simulink model "chap05"  (R2021a)
settings: Solver=FixedStepDiscrete  StartTime=0.0  StopTime=inf  FixedStep=0.001  RelTol=1e-3
undefined symbols (not defined in the file): DiscIntNeverNeededParam, Header, Pose, X, Y, Z
libraries: robotlib x31
(part 8 of 9)

== system chap05/Subsystem16/Subsystem2/Subsystem9/Subsystem ==
  switch : Inport
  zt3 : Inport  Port=2
  Constant4 : Constant  Value=0
  Discrete-Time Integrator : DiscreteIntegrator  SampleTime=-1  UpperSaturationLimit=100  LowerSaturationLimit=-100  ICPrevOutput=DiscIntNeverNeededParam  ICPrevScaledInput=DiscIntNeverNeededParam
  Logical Operator : Logic  AllPortsSameDT=off  OutDataTypeStr=boolean
  MATLAB Function : MATLAB Function  TreatAsAtomicUnit=on
  Relational Operator : RelationalOperator  Operator===  OutDataTypeStr=boolean  RndMeth=Simplest
  Saturation1 : Saturate  UpperLimit=0.25  LowerLimit=-0.25
  Sign : Signum
  Sign1 : Signum
  Subsystem : Subsystem
      settings: PortSchema="{\"entries\":[{\"content\":{\"sides\":[{\"content\":{\"connectorIds\":[\"In1\"]},\"type\":\"ConnectorPlacement.EquallySpacedRectSide\",\"uuid\":\"50b1559e-7173-4ba8-93e6-314f6d9df527\"},{\"content\":{\"connectorIds\":[\"Out1\"],\"side\":\"RIGHT\"},\"type\":\"ConnectorPlacement.EquallySpacedRectSide\",\"uuid\":\"be527bac-0bcc-4faf-a185-0382edae0189\"},{\"content\":{\"connectorIds\":[\"In2\"],\"side\":\"TOP\"},\"type\":\"ConnectorPlacement.EquallySpacedRectSide\",\"uuid\":\"4c8ef68d-7cf5-4d15-9758-89dbc1169805\"}]},\"type\":\"ConnectorPlacement.EquallySpacedConnector\",\"uuid\":\"3c2ee67b-c3c9-431a-8107-6d5cd22b236e\"}],\"packageUris\":[\"http://schema.mathworks.com/mf0/Connector/R2020b\"],\"version\":\"1.0\"}"
  Switch : Switch  Criteria=u2 > Threshold
  Out1 : Outport
  wires:
  zt3/1 -> Subsystem/1(zt3)
  switch/1 -> Subsystem/2(switch)
  Switch/1 -> Discrete-Time Integrator/1
  Logical Operator/1 -> Switch/2
  Sign/1 -> Relational Operator/2
  Discrete-Time Integrator/1 -> Saturation1/1, Sign/1, MATLAB Function/1(u1)
  Saturation1/1 -> MATLAB Function/2(u2), Out1/1
  Subsystem/1(Out1) -> Switch/3, Sign1/1
  Sign1/1 -> Relational Operator/1
  Constant4/1 -> Switch/1
  Relational Operator/1 -> Logical Operator/2
  MATLAB Function/1(y) -> Logical Operator/1

== system chap05/Subsystem16/Subsystem3/Subsystem11/Subsystem ==
  switch : Inport
  zt3 : Inport  Port=2
  Constant4 : Constant  Value=0
  Discrete-Time Integrator : DiscreteIntegrator  SampleTime=-1  UpperSaturationLimit=100  LowerSaturationLimit=-100  ICPrevOutput=DiscIntNeverNeededParam  ICPrevScaledInput=DiscIntNeverNeededParam
  Logical Operator : Logic  AllPortsSameDT=off  OutDataTypeStr=boolean
  MATLAB Function : MATLAB Function  TreatAsAtomicUnit=on
  Relational Operator : RelationalOperator  Operator===  OutDataTypeStr=boolean  RndMeth=Simplest
  Saturation1 : Saturate  UpperLimit=0.25  LowerLimit=-0.25
  Sign : Signum
  Sign1 : Signum
  Subsystem : Subsystem
      settings: PortSchema="{\"entries\":[{\"content\":{\"sides\":[{\"content\":{\"connectorIds\":[\"In1\"]},\"type\":\"ConnectorPlacement.EquallySpacedRectSide\",\"uuid\":\"50b1559e-7173-4ba8-93e6-314f6d9df527\"},{\"content\":{\"connectorIds\":[\"Out1\"],\"side\":\"RIGHT\"},\"type\":\"ConnectorPlacement.EquallySpacedRectSide\",\"uuid\":\"be527bac-0bcc-4faf-a185-0382edae0189\"},{\"content\":{\"connectorIds\":[\"In2\"],\"side\":\"TOP\"},\"type\":\"ConnectorPlacement.EquallySpacedRectSide\",\"uuid\":\"4c8ef68d-7cf5-4d15-9758-89dbc1169805\"}]},\"type\":\"ConnectorPlacement.EquallySpacedConnector\",\"uuid\":\"3c2ee67b-c3c9-431a-8107-6d5cd22b236e\"}],\"packageUris\":[\"http://schema.mathworks.com/mf0/Connector/R2020b\"],\"version\":\"1.0\"}"
  Switch : Switch  Criteria=u2 > Threshold
  Out1 : Outport
  wires:
  MATLAB Function/1(y) -> Logical Operator/1
  Relational Operator/1 -> Logical Operator/2
  Constant4/1 -> Switch/1
  Sign1/1 -> Relational Operator/1
  Subsystem/1(Out1) -> Sign1/1, Switch/3
  Saturation1/1 -> Out1/1, MATLAB Function/2(u2)
  Discrete-Time Integrator/1 -> Saturation1/1, MATLAB Function/1(u1), Sign/1
  Sign/1 -> Relational Operator/2
  Logical Operator/1 -> Switch/2
  Switch/1 -> Discrete-Time Integrator/1
  zt3/1 -> Subsystem/1(zt3)
  switch/1 -> Subsystem/2(switch)

== system chap05/Subsystem16/Subsystem3/Subsystem3/Subsystem ==
  e1 : Inport
  k3 : Inport  Port=2
  k4 : Inport  Port=3
  Add : Sum
  Constant3 : Constant  Value=-1
  Constant4 : Constant  Value=-1
  Discrete-Time Integrator1 : DiscreteIntegrator  SampleTime=-1  ICPrevOutput=DiscIntNeverNeededParam  ICPrevScaledInput=DiscIntNeverNeededParam
  Divide : Product  Inputs=*/
  MATLAB Function : MATLAB Function  TreatAsAtomicUnit=on
  Product3 : Product  Inputs=3
  Product5 : Product  Inputs=3
  z2 : Outport
  wires:
  Constant4/1 -> Product5/1
  Product5/1 -> Add/2
  Discrete-Time Integrator1/1 -> z2/1
  k3/1 -> Product3/3
  k4/1 -> Product5/3
  Divide/1 -> Add/1
  Add/1 -> Discrete-Time Integrator1/1
  Constant3/1 -> Product3/1
  e1/1 -> Product5/2, MATLAB Function/1(u), Product3/2
  MATLAB Function/1(y) -> Divide/2
  Product3/1 -> Divide/1

== system chap05/Subsystem16/Subsystem3/Subsystem3/Subsystem1 ==
  e1 : Inport
  k1 : Inport  Port=2
  Constant : Constant  Value=-1
  Divide : Product  Inputs=*/
  MATLAB Function : MATLAB Function  TreatAsAtomicUnit=on
  Product : Product  Inputs=3
  Out1 : Outport
  wires:
  e1/1 -> Product/2, MATLAB Function/1(u)
  Divide/1 -> Out1/1
  Constant/1 -> Product/1
  k1/1 -> Product/3
  MATLAB Function/1(y) -> Divide/2
  Product/1 -> Divide/1

== system chap05/Subsystem16/Subsystem3/Subsystem3/Subsystem2 ==
  e1 : Inport
  switch : Inport  Port=2
  Constant1 : Constant  Value=0.1
  MATLAB Function : MATLAB Function  TreatAsAtomicUnit=on
  Product{,1..3,6} (5 alike) : Product
  Sqrt : Sqrt  SaturateOnIntegerOverflow=on
  Square : Math  Operator=square  SaturateOnIntegerOverflow=on
  Subsystem : Subsystem
      settings: PortSchema="{\"entries\":[{\"content\":{\"sides\":[{\"content\":{\"connectorIds\":[\"In1\"]},\"type\":\"ConnectorPlacement.EquallySpacedRectSide\",\"uuid\":\"12a3f2f0-a297-420d-b26a-5f62088d5514\"},{\"content\":{\"connectorIds\":[\"Out1\"],\"side\":\"RIGHT\"},\"type\":\"ConnectorPlacement.EquallySpacedRectSide\",\"uuid\":\"62e35448-e0a3-4495-a6db-77deef7aa7b4\"},{\"content\":{\"connectorIds\":[\"In2\"],\"side\":\"TOP\"},\"type\":\"ConnectorPlacement.EquallySpacedRectSide\",\"uuid\":\"3e6c604a-b26b-4ac2-9bdc-2cdec7247e53\"}]},\"type\":\"ConnectorPlacement.EquallySpacedConnector\",\"uuid\":\"6331fe4a-63c7-4003-9b0d-be968a8635fa\"}],\"packageUris\":[\"http://schema.mathworks.com/mf0/Connector/R2020b\"],\"version\":\"1.0\"}"
  Subtract2 : Sum  Inputs=+-
  c1 : Constant  Value=0.1
  c2 : Constant  Value=0.1
  c3 : Constant  Value=0.3
  c4 : Constant  Value=0.3
  k1 : Outport
  k2 : Outport  Port=2
  k3 : Outport  Port=3
  k4 : Outport  Port=4
  wires:
  c2/1 -> Product/2
  Product/1 -> k2/1
  c3/1 -> Product1/1
  Product1/1 -> k3/1
  c4/1 -> Product2/1
  Product2/1 -> k4/1
  c1/1 -> Product3/2
  Product3/1 -> k1/1
  Sqrt/1 -> Product3/1
  Square/1 -> Product2/2
  e1/1 -> MATLAB Function/1(u)
  Product6/1 -> Subtract2/2
  MATLAB Function/1(y) -> Subtract2/1
  Subtract2/1 -> Subsystem/1(In1)
  Constant1/1 -> Product6/1
  switch/1 -> Subsystem/2(switch)
  Subsystem/1(Out1) -> Product6/2, Sqrt/1, Product1/2, Square/1, Product/1

== system chap05/Subsystem16/Subsystem3/Subsystem3/Subsystem3 ==
  e1 : Inport
  k2 : Inport  Port=2
  Constant2 : Constant  Value=-1
  Product2 : Product  Inputs=3
  Out1 : Outport
  wires:
  Product2/1 -> Out1/1
  e1/1 -> Product2/2
  k2/1 -> Product2/3
  Constant2/1 -> Product2/1

== system chap05/Subsystem16/Subsystem3/Subsystem4/Subsystem ==
  switch : Inport
  zt3 : Inport  Port=2
  Constant4 : Constant  Value=0
  Discrete-Time Integrator : DiscreteIntegrator  SampleTime=-1  UpperSaturationLimit=100  LowerSaturationLimit=-100  ICPrevOutput=DiscIntNeverNeededParam  ICPrevScaledInput=DiscIntNeverNeededParam
  Logical Operator : Logic  AllPortsSameDT=off  OutDataTypeStr=boolean
  MATLAB Function : MATLAB Function  TreatAsAtomicUnit=on
  Relational Operator : RelationalOperator  Operator===  OutDataTypeStr=boolean  RndMeth=Simplest
  Saturation1 : Saturate  UpperLimit=0.25  LowerLimit=-0.25
  Sign : Signum
  Sign1 : Signum
  Subsystem : Subsystem
      settings: PortSchema="{\"entries\":[{\"content\":{\"sides\":[{\"content\":{\"connectorIds\":[\"In1\"]},\"type\":\"ConnectorPlacement.EquallySpacedRectSide\",\"uuid\":\"50b1559e-7173-4ba8-93e6-314f6d9df527\"},{\"content\":{\"connectorIds\":[\"Out1\"],\"side\":\"RIGHT\"},\"type\":\"ConnectorPlacement.EquallySpacedRectSide\",\"uuid\":\"be527bac-0bcc-4faf-a185-0382edae0189\"},{\"content\":{\"connectorIds\":[\"In2\"],\"side\":\"TOP\"},\"type\":\"ConnectorPlacement.EquallySpacedRectSide\",\"uuid\":\"4c8ef68d-7cf5-4d15-9758-89dbc1169805\"}]},\"type\":\"ConnectorPlacement.EquallySpacedConnector\",\"uuid\":\"3c2ee67b-c3c9-431a-8107-6d5cd22b236e\"}],\"packageUris\":[\"http://schema.mathworks.com/mf0/Connector/R2020b\"],\"version\":\"1.0\"}"
  Switch : Switch  Criteria=u2 > Threshold
  Out1 : Outport
  wires:
  MATLAB Function/1(y) -> Logical Operator/1
  Relational Operator/1 -> Logical Operator/2
  Constant4/1 -> Switch/1
  Sign1/1 -> Relational Operator/1
  Subsystem/1(Out1) -> Sign1/1, Switch/3
  Saturation1/1 -> Out1/1, MATLAB Function/2(u2)
  Discrete-Time Integrator/1 -> Saturation1/1, MATLAB Function/1(u1), Sign/1
  Sign/1 -> Relational Operator/2
  Logical Operator/1 -> Switch/2
  Switch/1 -> Discrete-Time Integrator/1
  zt3/1 -> Subsystem/1(zt3)
  switch/1 -> Subsystem/2(switch)

== system chap05/Subsystem16/Subsystem3/Subsystem8/Subsystem ==
  In1 : Inport
  switch : Inport  Port=2
  Constant4 : Constant  Value=0
  Switch1 : Switch  Criteria=u2 > Threshold
  Out1 : Outport
  wires:
  In1/1 -> Switch1/1
  Switch1/1 -> Out1/1
  switch/1 -> Switch1/2
  Constant4/1 -> Switch1/3

== system chap05/Subsystem16/Subsystem3/Subsystem8/Subsystem1 ==
  In1 : Inport
  switch : Inport  Port=2
  Constant4 : Constant  Value=0
  Switch1 : Switch  Criteria=u2 > Threshold
  Out1 : Outport
  wires:
  Constant4/1 -> Switch1/3
  switch/1 -> Switch1/2
  Switch1/1 -> Out1/1
  In1/1 -> Switch1/1

== system chap05/Subsystem16/Subsystem3/Subsystem8/Subsystem2 ==
  In1 : Inport
  switch : Inport  Port=2
  Constant4 : Constant  Value=0
  Switch1 : Switch  Criteria=u2 > Threshold
  Out1 : Outport
  wires:
  In1/1 -> Switch1/1
  Switch1/1 -> Out1/1
  switch/1 -> Switch1/2
  Constant4/1 -> Switch1/3

== system chap05/Subsystem16/Subsystem3/Subsystem9/Subsystem ==
  switch : Inport
  zt3 : Inport  Port=2
  Constant4 : Constant  Value=0
  Discrete-Time Integrator : DiscreteIntegrator  SampleTime=-1  UpperSaturationLimit=100  LowerSaturationLimit=-100  ICPrevOutput=DiscIntNeverNeededParam  ICPrevScaledInput=DiscIntNeverNeededParam
  Logical Operator : Logic  AllPortsSameDT=off  OutDataTypeStr=boolean
  MATLAB Function : MATLAB Function  TreatAsAtomicUnit=on
  Relational Operator : RelationalOperator  Operator===  OutDataTypeStr=boolean  RndMeth=Simplest
  Saturation1 : Saturate  UpperLimit=0.25  LowerLimit=-0.25
  Sign : Signum
  Sign1 : Signum
  Subsystem : Subsystem
      settings: PortSchema="{\"entries\":[{\"content\":{\"sides\":[{\"content\":{\"connectorIds\":[\"In1\"]},\"type\":\"ConnectorPlacement.EquallySpacedRectSide\",\"uuid\":\"50b1559e-7173-4ba8-93e6-314f6d9df527\"},{\"content\":{\"connectorIds\":[\"Out1\"],\"side\":\"RIGHT\"},\"type\":\"ConnectorPlacement.EquallySpacedRectSide\",\"uuid\":\"be527bac-0bcc-4faf-a185-0382edae0189\"},{\"content\":{\"connectorIds\":[\"In2\"],\"side\":\"TOP\"},\"type\":\"ConnectorPlacement.EquallySpacedRectSide\",\"uuid\":\"4c8ef68d-7cf5-4d15-9758-89dbc1169805\"}]},\"type\":\"ConnectorPlacement.EquallySpacedConnector\",\"uuid\":\"3c2ee67b-c3c9-431a-8107-6d5cd22b236e\"}],\"packageUris\":[\"http://schema.mathworks.com/mf0/Connector/R2020b\"],\"version\":\"1.0\"}"
  Switch : Switch  Criteria=u2 > Threshold
  Out1 : Outport
  wires:
  zt3/1 -> Subsystem/1(zt3)
  switch/1 -> Subsystem/2(switch)
  Switch/1 -> Discrete-Time Integrator/1
  Logical Operator/1 -> Switch/2
  Sign/1 -> Relational Operator/2
  Discrete-Time Integrator/1 -> Saturation1/1, Sign/1, MATLAB Function/1(u1)
  Saturation1/1 -> MATLAB Function/2(u2), Out1/1
  Subsystem/1(Out1) -> Switch/3, Sign1/1
  Sign1/1 -> Relational Operator/1
  Constant4/1 -> Switch/1
  Relational Operator/1 -> Logical Operator/2
  MATLAB Function/1(y) -> Logical Operator/1

== system chap05/Subsystem16/Subsystem5/Subsystem11/Subsystem ==
  switch : Inport
  zt3 : Inport  Port=2
  Constant4 : Constant  Value=0
  Discrete-Time Integrator : DiscreteIntegrator  SampleTime=-1  UpperSaturationLimit=100  LowerSaturationLimit=-100  ICPrevOutput=DiscIntNeverNeededParam  ICPrevScaledInput=DiscIntNeverNeededParam
  Logical Operator : Logic  AllPortsSameDT=off  OutDataTypeStr=boolean
  MATLAB Function : MATLAB Function  TreatAsAtomicUnit=on
  Relational Operator : RelationalOperator  Operator===  OutDataTypeStr=boolean  RndMeth=Simplest
  Saturation1 : Saturate  UpperLimit=0.25  LowerLimit=-0.25
  Sign : Signum
  Sign1 : Signum
  Subsystem : Subsystem
      settings: PortSchema="{\"entries\":[{\"content\":{\"sides\":[{\"content\":{\"connectorIds\":[\"In1\"]},\"type\":\"ConnectorPlacement.EquallySpacedRectSide\",\"uuid\":\"50b1559e-7173-4ba8-93e6-314f6d9df527\"},{\"content\":{\"connectorIds\":[\"Out1\"],\"side\":\"RIGHT\"},\"type\":\"ConnectorPlacement.EquallySpacedRectSide\",\"uuid\":\"be527bac-0bcc-4faf-a185-0382edae0189\"},{\"content\":{\"connectorIds\":[\"In2\"],\"side\":\"TOP\"},\"type\":\"ConnectorPlacement.EquallySpacedRectSide\",\"uuid\":\"4c8ef68d-7cf5-4d15-9758-89dbc1169805\"}]},\"type\":\"ConnectorPlacement.EquallySpacedConnector\",\"uuid\":\"3c2ee67b-c3c9-431a-8107-6d5cd22b236e\"}],\"packageUris\":[\"http://schema.mathworks.com/mf0/Connector/R2020b\"],\"version\":\"1.0\"}"
  Switch : Switch  Criteria=u2 > Threshold
  Out1 : Outport
  wires:
  MATLAB Function/1(y) -> Logical Operator/1
  Relational Operator/1 -> Logical Operator/2
  Constant4/1 -> Switch/1
  Sign1/1 -> Relational Operator/1
  Subsystem/1(Out1) -> Sign1/1, Switch/3
  Saturation1/1 -> Out1/1, MATLAB Function/2(u2)
  Discrete-Time Integrator/1 -> Saturation1/1, MATLAB Function/1(u1), Sign/1
  Sign/1 -> Relational Operator/2
  Logical Operator/1 -> Switch/2
  Switch/1 -> Discrete-Time Integrator/1
  zt3/1 -> Subsystem/1(zt3)
  switch/1 -> Subsystem/2(switch)

== system chap05/Subsystem16/Subsystem5/Subsystem3/Subsystem ==
  e1 : Inport
  k3 : Inport  Port=2
  k4 : Inport  Port=3
  Add : Sum
  Constant3 : Constant  Value=-1
  Constant4 : Constant  Value=-1
  Discrete-Time Integrator1 : DiscreteIntegrator  SampleTime=-1  ICPrevOutput=DiscIntNeverNeededParam  ICPrevScaledInput=DiscIntNeverNeededParam
  Divide : Product  Inputs=*/
  MATLAB Function : MATLAB Function  TreatAsAtomicUnit=on
  Product3 : Product  Inputs=3
  Product5 : Product  Inputs=3
  z2 : Outport
  wires:
  Constant4/1 -> Product5/1
  Product5/1 -> Add/2
  Discrete-Time Integrator1/1 -> z2/1
  k3/1 -> Product3/3
  k4/1 -> Product5/3
  Divide/1 -> Add/1
  Add/1 -> Discrete-Time Integrator1/1
  Constant3/1 -> Product3/1
  e1/1 -> Product5/2, MATLAB Function/1(u), Product3/2
  MATLAB Function/1(y) -> Divide/2
  Product3/1 -> Divide/1

== system chap05/Subsystem16/Subsystem5/Subsystem3/Subsystem1 ==
  e1 : Inport
  k1 : Inport  Port=2
  Constant : Constant  Value=-1
  Divide : Product  Inputs=*/
  MATLAB Function : MATLAB Function  TreatAsAtomicUnit=on
  Product : Product  Inputs=3
  Out1 : Outport
  wires:
  e1/1 -> Product/2, MATLAB Function/1(u)
  Divide/1 -> Out1/1
  Constant/1 -> Product/1
  k1/1 -> Product/3
  MATLAB Function/1(y) -> Divide/2
  Product/1 -> Divide/1

== system chap05/Subsystem16/Subsystem5/Subsystem3/Subsystem2 ==
  e1 : Inport
  switch : Inport  Port=2
  Constant1 : Constant  Value=0.1
  MATLAB Function : MATLAB Function  TreatAsAtomicUnit=on
  Product{,1..3,6} (5 alike) : Product
  Sqrt : Sqrt  SaturateOnIntegerOverflow=on
  Square : Math  Operator=square  SaturateOnIntegerOverflow=on
  Subsystem : Subsystem
      settings: PortSchema="{\"entries\":[{\"content\":{\"sides\":[{\"content\":{\"connectorIds\":[\"In1\"]},\"type\":\"ConnectorPlacement.EquallySpacedRectSide\",\"uuid\":\"12a3f2f0-a297-420d-b26a-5f62088d5514\"},{\"content\":{\"connectorIds\":[\"Out1\"],\"side\":\"RIGHT\"},\"type\":\"ConnectorPlacement.EquallySpacedRectSide\",\"uuid\":\"62e35448-e0a3-4495-a6db-77deef7aa7b4\"},{\"content\":{\"connectorIds\":[\"In2\"],\"side\":\"TOP\"},\"type\":\"ConnectorPlacement.EquallySpacedRectSide\",\"uuid\":\"3e6c604a-b26b-4ac2-9bdc-2cdec7247e53\"}]},\"type\":\"ConnectorPlacement.EquallySpacedConnector\",\"uuid\":\"6331fe4a-63c7-4003-9b0d-be968a8635fa\"}],\"packageUris\":[\"http://schema.mathworks.com/mf0/Connector/R2020b\"],\"version\":\"1.0\"}"
  Subtract2 : Sum  Inputs=+-
  c1 : Constant  Value=0.1
  c2 : Constant  Value=0.1
  c3 : Constant  Value=0.3
  c4 : Constant  Value=0.3
  k1 : Outport
  k2 : Outport  Port=2
  k3 : Outport  Port=3
  k4 : Outport  Port=4
  wires:
  c2/1 -> Product/2
  Product/1 -> k2/1
  c3/1 -> Product1/1
  Product1/1 -> k3/1
  c4/1 -> Product2/1
  Product2/1 -> k4/1
  c1/1 -> Product3/2
  Product3/1 -> k1/1
  Sqrt/1 -> Product3/1
  Square/1 -> Product2/2
  e1/1 -> MATLAB Function/1(u)
  Product6/1 -> Subtract2/2
  MATLAB Function/1(y) -> Subtract2/1
  Subtract2/1 -> Subsystem/1(In1)
  Constant1/1 -> Product6/1
  switch/1 -> Subsystem/2(switch)
  Subsystem/1(Out1) -> Product6/2, Sqrt/1, Product1/2, Square/1, Product/1

== system chap05/Subsystem16/Subsystem5/Subsystem3/Subsystem3 ==
  e1 : Inport
  k2 : Inport  Port=2
  Constant2 : Constant  Value=-1
  Product2 : Product  Inputs=3
  Out1 : Outport
  wires:
  Product2/1 -> Out1/1
  e1/1 -> Product2/2
  k2/1 -> Product2/3
  Constant2/1 -> Product2/1

== system chap05/Subsystem16/Subsystem5/Subsystem4/Subsystem ==
  switch : Inport
  zt3 : Inport  Port=2
  Constant4 : Constant  Value=0
  Discrete-Time Integrator : DiscreteIntegrator  SampleTime=-1  UpperSaturationLimit=100  LowerSaturationLimit=-100  ICPrevOutput=DiscIntNeverNeededParam  ICPrevScaledInput=DiscIntNeverNeededParam
  Logical Operator : Logic  AllPortsSameDT=off  OutDataTypeStr=boolean
  MATLAB Function : MATLAB Function  TreatAsAtomicUnit=on
  Relational Operator : RelationalOperator  Operator===  OutDataTypeStr=boolean  RndMeth=Simplest
  Saturation1 : Saturate  UpperLimit=0.25  LowerLimit=-0.25
  Sign : Signum
  Sign1 : Signum
  Subsystem : Subsystem
      settings: PortSchema="{\"entries\":[{\"content\":{\"sides\":[{\"content\":{\"connectorIds\":[\"In1\"]},\"type\":\"ConnectorPlacement.EquallySpacedRectSide\",\"uuid\":\"50b1559e-7173-4ba8-93e6-314f6d9df527\"},{\"content\":{\"connectorIds\":[\"Out1\"],\"side\":\"RIGHT\"},\"type\":\"ConnectorPlacement.EquallySpacedRectSide\",\"uuid\":\"be527bac-0bcc-4faf-a185-0382edae0189\"},{\"content\":{\"connectorIds\":[\"In2\"],\"side\":\"TOP\"},\"type\":\"ConnectorPlacement.EquallySpacedRectSide\",\"uuid\":\"4c8ef68d-7cf5-4d15-9758-89dbc1169805\"}]},\"type\":\"ConnectorPlacement.EquallySpacedConnector\",\"uuid\":\"3c2ee67b-c3c9-431a-8107-6d5cd22b236e\"}],\"packageUris\":[\"http://schema.mathworks.com/mf0/Connector/R2020b\"],\"version\":\"1.0\"}"
  Switch : Switch  Criteria=u2 > Threshold
  Out1 : Outport
  wires:
  MATLAB Function/1(y) -> Logical Operator/1
  Relational Operator/1 -> Logical Operator/2
  Constant4/1 -> Switch/1
  Sign1/1 -> Relational Operator/1
  Subsystem/1(Out1) -> Sign1/1, Switch/3
  Saturation1/1 -> Out1/1, MATLAB Function/2(u2)
  Discrete-Time Integrator/1 -> Saturation1/1, MATLAB Function/1(u1), Sign/1
  Sign/1 -> Relational Operator/2
  Logical Operator/1 -> Switch/2
  Switch/1 -> Discrete-Time Integrator/1
  zt3/1 -> Subsystem/1(zt3)
  switch/1 -> Subsystem/2(switch)

== system chap05/Subsystem16/Subsystem5/Subsystem7/Subsystem ==
  In1 : Inport
  switch : Inport  Port=2
  Constant4 : Constant  Value=0
  Switch1 : Switch  Criteria=u2 > Threshold
  Out1 : Outport
  wires:
  In1/1 -> Switch1/1
  Switch1/1 -> Out1/1
  switch/1 -> Switch1/2
  Constant4/1 -> Switch1/3

== system chap05/Subsystem16/Subsystem5/Subsystem7/Subsystem1 ==
  In1 : Inport
  switch : Inport  Port=2
  Constant4 : Constant  Value=0
  Switch1 : Switch  Criteria=u2 > Threshold
  Out1 : Outport
  wires:
  Constant4/1 -> Switch1/3
  switch/1 -> Switch1/2
  Switch1/1 -> Out1/1
  In1/1 -> Switch1/1

== system chap05/Subsystem16/Subsystem5/Subsystem7/Subsystem2 ==
  In1 : Inport
  switch : Inport  Port=2
  Constant4 : Constant  Value=0
  Switch1 : Switch  Criteria=u2 > Threshold
  Out1 : Outport
  wires:
  In1/1 -> Switch1/1
  Switch1/1 -> Out1/1
  switch/1 -> Switch1/2
  Constant4/1 -> Switch1/3

== system chap05/Subsystem16/Subsystem5/Subsystem9/Subsystem ==
  switch : Inport
  zt3 : Inport  Port=2
  Constant4 : Constant  Value=0
  Discrete-Time Integrator : DiscreteIntegrator  SampleTime=-1  UpperSaturationLimit=100  LowerSaturationLimit=-100  ICPrevOutput=DiscIntNeverNeededParam  ICPrevScaledInput=DiscIntNeverNeededParam
  Logical Operator : Logic  AllPortsSameDT=off  OutDataTypeStr=boolean
  MATLAB Function : MATLAB Function  TreatAsAtomicUnit=on
  Relational Operator : RelationalOperator  Operator===  OutDataTypeStr=boolean  RndMeth=Simplest
  Saturation1 : Saturate  UpperLimit=0.25  LowerLimit=-0.25
  Sign : Signum
  Sign1 : Signum
  Subsystem : Subsystem
      settings: PortSchema="{\"entries\":[{\"content\":{\"sides\":[{\"content\":{\"connectorIds\":[\"In1\"]},\"type\":\"ConnectorPlacement.EquallySpacedRectSide\",\"uuid\":\"50b1559e-7173-4ba8-93e6-314f6d9df527\"},{\"content\":{\"connectorIds\":[\"Out1\"],\"side\":\"RIGHT\"},\"type\":\"ConnectorPlacement.EquallySpacedRectSide\",\"uuid\":\"be527bac-0bcc-4faf-a185-0382edae0189\"},{\"content\":{\"connectorIds\":[\"In2\"],\"side\":\"TOP\"},\"type\":\"ConnectorPlacement.EquallySpacedRectSide\",\"uuid\":\"4c8ef68d-7cf5-4d15-9758-89dbc1169805\"}]},\"type\":\"ConnectorPlacement.EquallySpacedConnector\",\"uuid\":\"3c2ee67b-c3c9-431a-8107-6d5cd22b236e\"}],\"packageUris\":[\"http://schema.mathworks.com/mf0/Connector/R2020b\"],\"version\":\"1.0\"}"
  Switch : Switch  Criteria=u2 > Threshold
  Out1 : Outport
  wires:
  zt3/1 -> Subsystem/1(zt3)
  switch/1 -> Subsystem/2(switch)
  Switch/1 -> Discrete-Time Integrator/1
  Logical Operator/1 -> Switch/2
  Sign/1 -> Relational Operator/2
  Discrete-Time Integrator/1 -> Saturation1/1, Sign/1, MATLAB Function/1(u1)
  Saturation1/1 -> MATLAB Function/2(u2), Out1/1
  Subsystem/1(Out1) -> Switch/3, Sign1/1
  Sign1/1 -> Relational Operator/1
  Constant4/1 -> Switch/1
  Relational Operator/1 -> Logical Operator/2
  MATLAB Function/1(y) -> Logical Operator/1

== system chap05/Subsystem16/Subsystem6/Subsystem3/Subsystem ==
  e1 : Inport
  k3 : Inport  Port=2
  k4 : Inport  Port=3
  Add : Sum
  Constant3 : Constant  Value=-1
  Constant4 : Constant  Value=-1
  Discrete-Time Integrator1 : DiscreteIntegrator  SampleTime=-1  ICPrevOutput=DiscIntNeverNeededParam  ICPrevScaledInput=DiscIntNeverNeededParam
  Divide : Product  Inputs=*/
  MATLAB Function : MATLAB Function  TreatAsAtomicUnit=on
  Product3 : Product  Inputs=3
  Product5 : Product  Inputs=3
  z2 : Outport
  wires:
  Constant4/1 -> Product5/1
  Product5/1 -> Add/2
  Discrete-Time Integrator1/1 -> z2/1
  k3/1 -> Product3/3
  k4/1 -> Product5/3
  Divide/1 -> Add/1
  Add/1 -> Discrete-Time Integrator1/1
  Constant3/1 -> Product3/1
  e1/1 -> Product5/2, MATLAB Function/1(u), Product3/2
  MATLAB Function/1(y) -> Divide/2
  Product3/1 -> Divide/1

== system chap05/Subsystem16/Subsystem6/Subsystem3/Subsystem1 ==
  e1 : Inport
  k1 : Inport  Port=2
  Constant : Constant  Value=-1
  Divide : Product  Inputs=*/
  MATLAB Function : MATLAB Function  TreatAsAtomicUnit=on
  Product : Product  Inputs=3
  Out1 : Outport
  wires:
  e1/1 -> Product/2, MATLAB Function/1(u)
  Divide/1 -> Out1/1
  Constant/1 -> Product/1
  k1/1 -> Product/3
  MATLAB Function/1(y) -> Divide/2
  Product/1 -> Divide/1

== system chap05/Subsystem16/Subsystem6/Subsystem3/Subsystem2 ==
  e1 : Inport
  switch : Inport  Port=2
  Constant1 : Constant  Value=0.1
  MATLAB Function : MATLAB Function  TreatAsAtomicUnit=on
  Product{,1..3,6} (5 alike) : Product
  Sqrt : Sqrt  SaturateOnIntegerOverflow=on
  Square : Math  Operator=square  SaturateOnIntegerOverflow=on
  Subsystem : Subsystem
      settings: PortSchema="{\"entries\":[{\"content\":{\"sides\":[{\"content\":{\"connectorIds\":[\"In1\"]},\"type\":\"ConnectorPlacement.EquallySpacedRectSide\",\"uuid\":\"12a3f2f0-a297-420d-b26a-5f62088d5514\"},{\"content\":{\"connectorIds\":[\"Out1\"],\"side\":\"RIGHT\"},\"type\":\"ConnectorPlacement.EquallySpacedRectSide\",\"uuid\":\"62e35448-e0a3-4495-a6db-77deef7aa7b4\"},{\"content\":{\"connectorIds\":[\"In2\"],\"side\":\"TOP\"},\"type\":\"ConnectorPlacement.EquallySpacedRectSide\",\"uuid\":\"3e6c604a-b26b-4ac2-9bdc-2cdec7247e53\"}]},\"type\":\"ConnectorPlacement.EquallySpacedConnector\",\"uuid\":\"6331fe4a-63c7-4003-9b0d-be968a8635fa\"}],\"packageUris\":[\"http://schema.mathworks.com/mf0/Connector/R2020b\"],\"version\":\"1.0\"}"
  Subtract2 : Sum  Inputs=+-
  c1 : Constant  Value=0.1
  c2 : Constant  Value=0.1
  c3 : Constant  Value=0.3
  c4 : Constant  Value=0.3
  k1 : Outport
  k2 : Outport  Port=2
  k3 : Outport  Port=3
  k4 : Outport  Port=4
  wires:
  c2/1 -> Product/2
  Product/1 -> k2/1
  c3/1 -> Product1/1
  Product1/1 -> k3/1
  c4/1 -> Product2/1
  Product2/1 -> k4/1
  c1/1 -> Product3/2
  Product3/1 -> k1/1
  Sqrt/1 -> Product3/1
  Square/1 -> Product2/2
  e1/1 -> MATLAB Function/1(u)
  Product6/1 -> Subtract2/2
  MATLAB Function/1(y) -> Subtract2/1
  Subtract2/1 -> Subsystem/1(In1)
  Constant1/1 -> Product6/1
  switch/1 -> Subsystem/2(switch)
  Subsystem/1(Out1) -> Product6/2, Sqrt/1, Product1/2, Square/1, Product/1

== system chap05/Subsystem16/Subsystem6/Subsystem3/Subsystem3 ==
  e1 : Inport
  k2 : Inport  Port=2
  Constant2 : Constant  Value=-1
  Product2 : Product  Inputs=3
  Out1 : Outport
  wires:
  Product2/1 -> Out1/1
  e1/1 -> Product2/2
  k2/1 -> Product2/3
  Constant2/1 -> Product2/1

== system chap05/Subsystem16/Subsystem6/Subsystem4/Subsystem ==
  switch : Inport
  zt3 : Inport  Port=2
  Constant4 : Constant  Value=0
  Discrete-Time Integrator : DiscreteIntegrator  SampleTime=-1  UpperSaturationLimit=100  LowerSaturationLimit=-100  ICPrevOutput=DiscIntNeverNeededParam  ICPrevScaledInput=DiscIntNeverNeededParam
  Logical Operator : Logic  AllPortsSameDT=off  OutDataTypeStr=boolean
  MATLAB Function : MATLAB Function  TreatAsAtomicUnit=on
  Relational Operator : RelationalOperator  Operator===  OutDataTypeStr=boolean  RndMeth=Simplest
  Saturation1 : Saturate  UpperLimit=0.25  LowerLimit=-0.25
  Sign : Signum
  Sign1 : Signum
  Subsystem : Subsystem
      settings: PortSchema="{\"entries\":[{\"content\":{\"sides\":[{\"content\":{\"connectorIds\":[\"In1\"]},\"type\":\"ConnectorPlacement.EquallySpacedRectSide\",\"uuid\":\"50b1559e-7173-4ba8-93e6-314f6d9df527\"},{\"content\":{\"connectorIds\":[\"Out1\"],\"side\":\"RIGHT\"},\"type\":\"ConnectorPlacement.EquallySpacedRectSide\",\"uuid\":\"be527bac-0bcc-4faf-a185-0382edae0189\"},{\"content\":{\"connectorIds\":[\"In2\"],\"side\":\"TOP\"},\"type\":\"ConnectorPlacement.EquallySpacedRectSide\",\"uuid\":\"4c8ef68d-7cf5-4d15-9758-89dbc1169805\"}]},\"type\":\"ConnectorPlacement.EquallySpacedConnector\",\"uuid\":\"3c2ee67b-c3c9-431a-8107-6d5cd22b236e\"}],\"packageUris\":[\"http://schema.mathworks.com/mf0/Connector/R2020b\"],\"version\":\"1.0\"}"
  Switch : Switch  Criteria=u2 > Threshold
  Out1 : Outport
  wires:
  MATLAB Function/1(y) -> Logical Operator/1
  Relational Operator/1 -> Logical Operator/2
  Constant4/1 -> Switch/1
  Sign1/1 -> Relational Operator/1
  Subsystem/1(Out1) -> Sign1/1, Switch/3
  Saturation1/1 -> Out1/1, MATLAB Function/2(u2)
  Discrete-Time Integrator/1 -> Saturation1/1, MATLAB Function/1(u1), Sign/1
  Sign/1 -> Relational Operator/2
  Logical Operator/1 -> Switch/2
  Switch/1 -> Discrete-Time Integrator/1
  zt3/1 -> Subsystem/1(zt3)
  switch/1 -> Subsystem/2(switch)

== system chap05/Subsystem16/Subsystem6/Subsystem5/Subsystem ==
  switch : Inport
  zt3 : Inport  Port=2
  Constant4 : Constant  Value=0
  Discrete-Time Integrator : DiscreteIntegrator  SampleTime=-1  UpperSaturationLimit=100  LowerSaturationLimit=-100  ICPrevOutput=DiscIntNeverNeededParam  ICPrevScaledInput=DiscIntNeverNeededParam
  Logical Operator : Logic  AllPortsSameDT=off  OutDataTypeStr=boolean
  MATLAB Function : MATLAB Function  TreatAsAtomicUnit=on
  Relational Operator : RelationalOperator  Operator===  OutDataTypeStr=boolean  RndMeth=Simplest
  Saturation1 : Saturate  UpperLimit=0.25  LowerLimit=-0.25
  Sign : Signum
  Sign1 : Signum
  Subsystem : Subsystem
      settings: PortSchema="{\"entries\":[{\"content\":{\"sides\":[{\"content\":{\"connectorIds\":[\"In1\"]},\"type\":\"ConnectorPlacement.EquallySpacedRectSide\",\"uuid\":\"50b1559e-7173-4ba8-93e6-314f6d9df527\"},{\"content\":{\"connectorIds\":[\"Out1\"],\"side\":\"RIGHT\"},\"type\":\"ConnectorPlacement.EquallySpacedRectSide\",\"uuid\":\"be527bac-0bcc-4faf-a185-0382edae0189\"},{\"content\":{\"connectorIds\":[\"In2\"],\"side\":\"TOP\"},\"type\":\"ConnectorPlacement.EquallySpacedRectSide\",\"uuid\":\"4c8ef68d-7cf5-4d15-9758-89dbc1169805\"}]},\"type\":\"ConnectorPlacement.EquallySpacedConnector\",\"uuid\":\"3c2ee67b-c3c9-431a-8107-6d5cd22b236e\"}],\"packageUris\":[\"http://schema.mathworks.com/mf0/Connector/R2020b\"],\"version\":\"1.0\"}"
  Switch : Switch  Criteria=u2 > Threshold
  Out1 : Outport
  wires:
  zt3/1 -> Subsystem/1(zt3)
  switch/1 -> Subsystem/2(switch)
  Switch/1 -> Discrete-Time Integrator/1
  Logical Operator/1 -> Switch/2
  Sign/1 -> Relational Operator/2
  Discrete-Time Integrator/1 -> Saturation1/1, Sign/1, MATLAB Function/1(u1)
  Saturation1/1 -> MATLAB Function/2(u2), Out1/1
  Subsystem/1(Out1) -> Switch/3, Sign1/1
  Sign1/1 -> Relational Operator/1
  Constant4/1 -> Switch/1
  Relational Operator/1 -> Logical Operator/2
  MATLAB Function/1(y) -> Logical Operator/1

== system chap05/Subsystem16/Subsystem6/Subsystem7/Subsystem ==
  switch : Inport
  zt3 : Inport  Port=2
  Constant4 : Constant  Value=0
  Discrete-Time Integrator : DiscreteIntegrator  SampleTime=-1  UpperSaturationLimit=100  LowerSaturationLimit=-100  ICPrevOutput=DiscIntNeverNeededParam  ICPrevScaledInput=DiscIntNeverNeededParam
  Logical Operator : Logic  AllPortsSameDT=off  OutDataTypeStr=boolean
  MATLAB Function : MATLAB Function  TreatAsAtomicUnit=on
  Relational Operator : RelationalOperator  Operator===  OutDataTypeStr=boolean  RndMeth=Simplest
  Saturation1 : Saturate  UpperLimit=0.25  LowerLimit=-0.25
  Sign : Signum
  Sign1 : Signum
  Subsystem : Subsystem
      settings: PortSchema="{\"entries\":[{\"content\":{\"sides\":[{\"content\":{\"connectorIds\":[\"In1\"]},\"type\":\"ConnectorPlacement.EquallySpacedRectSide\",\"uuid\":\"50b1559e-7173-4ba8-93e6-314f6d9df527\"},{\"content\":{\"connectorIds\":[\"Out1\"],\"side\":\"RIGHT\"},\"type\":\"ConnectorPlacement.EquallySpacedRectSide\",\"uuid\":\"be527bac-0bcc-4faf-a185-0382edae0189\"},{\"content\":{\"connectorIds\":[\"In2\"],\"side\":\"TOP\"},\"type\":\"ConnectorPlacement.EquallySpacedRectSide\",\"uuid\":\"4c8ef68d-7cf5-4d15-9758-89dbc1169805\"}]},\"type\":\"ConnectorPlacement.EquallySpacedConnector\",\"uuid\":\"3c2ee67b-c3c9-431a-8107-6d5cd22b236e\"}],\"packageUris\":[\"http://schema.mathworks.com/mf0/Connector/R2020b\"],\"version\":\"1.0\"}"
  Switch : Switch  Criteria=u2 > Threshold
  Out1 : Outport
  wires:
  MATLAB Function/1(y) -> Logical Operator/1
  Relational Operator/1 -> Logical Operator/2
  Constant4/1 -> Switch/1
  Sign1/1 -> Relational Operator/1
  Subsystem/1(Out1) -> Sign1/1, Switch/3
  Saturation1/1 -> Out1/1, MATLAB Function/2(u2)
  Discrete-Time Integrator/1 -> Saturation1/1, MATLAB Function/1(u1), Sign/1
  Sign/1 -> Relational Operator/2
  Logical Operator/1 -> Switch/2
  Switch/1 -> Discrete-Time Integrator/1
  zt3/1 -> Subsystem/1(zt3)
  switch/1 -> Subsystem/2(switch)

== system chap05/Subsystem16/Subsystem6/Subsystem8/Subsystem ==
  In1 : Inport
  switch : Inport  Port=2
  Constant4 : Constant  Value=0
  Switch1 : Switch  Criteria=u2 > Threshold
  Out1 : Outport
  wires:
  In1/1 -> Switch1/1
  Switch1/1 -> Out1/1
  switch/1 -> Switch1/2
  Constant4/1 -> Switch1/3

== system chap05/Subsystem16/Subsystem6/Subsystem8/Subsystem1 ==
  In1 : Inport
  switch : Inport  Port=2
  Constant4 : Constant  Value=0
  Switch1 : Switch  Criteria=u2 > Threshold
  Out1 : Outport
  wires:
  Constant4/1 -> Switch1/3
  switch/1 -> Switch1/2
  Switch1/1 -> Out1/1
  In1/1 -> Switch1/1

== system chap05/Subsystem16/Subsystem6/Subsystem8/Subsystem2 ==
  In1 : Inport
  switch : Inport  Port=2
  Constant4 : Constant  Value=0
  Switch1 : Switch  Criteria=u2 > Threshold
  Out1 : Outport
  wires:
  In1/1 -> Switch1/1
  Switch1/1 -> Out1/1
  switch/1 -> Switch1/2
  Constant4/1 -> Switch1/3

== system chap05/Subsystem16/Subsystem/Subsystem11/Subsystem/Subsystem ==
  zt3 : Inport
  switch : Inport  Port=2
  Constant4 : Constant  Value=0
  Switch1 : Switch  Criteria=u2 > Threshold
  Out1 : Outport
  wires:
  Constant4/1 -> Switch1/3
  switch/1 -> Switch1/2
  Switch1/1 -> Out1/1
  zt3/1 -> Switch1/1

== system chap05/Subsystem16/Subsystem/Subsystem3/Subsystem2/Subsystem ==
  In1 : Inport
  switch : Inport  Port=2
  Constant1 : Constant  Value=0
  Constant2 : Constant  Value=0
  Discrete-Time Integrator2 : DiscreteIntegrator  gainval=1  InitialCondition=0.1  SampleTime=-1  ICPrevOutput=DiscIntNeverNeededParam  ICPrevScaledInput=DiscIntNeverNeededParam
  Switch : Switch  Criteria=u2 > Threshold
  Switch1 : Switch  Criteria=u2 > Threshold
  Out1 : Outport
  wires:
  switch/1 -> Switch/2, Switch1/2
  Switch1/1 -> Out1/1
  Constant2/1 -> Switch1/3
  Constant1/1 -> Switch/3
  Discrete-Time Integrator2/1 -> Switch1/1
  In1/1 -> Switch/1
  Switch/1 -> Discrete-Time Integrator2/1

== system chap05/Subsystem16/Subsystem/Subsystem4/Subsystem/Subsystem ==
  zt3 : Inport
  switch : Inport  Port=2
  Constant4 : Constant  Value=0
  Switch1 : Switch  Criteria=u2 > Threshold
  Out1 : Outport
  wires:
  Constant4/1 -> Switch1/3
  switch/1 -> Switch1/2
  Switch1/1 -> Out1/1
  zt3/1 -> Switch1/1

== system chap05/Subsystem16/Subsystem/Subsystem9/Subsystem/Subsystem ==
  zt3 : Inport
  switch : Inport  Port=2
  Constant4 : Constant  Value=0
  Switch1 : Switch  Criteria=u2 > Threshold
  Out1 : Outport
  wires:
  Constant4/1 -> Switch1/3
  switch/1 -> Switch1/2
  Switch1/1 -> Out1/1
  zt3/1 -> Switch1/1

== system chap05/Subsystem16/Subsystem1/Subsystem11/Subsystem/Subsystem ==
  zt3 : Inport
  switch : Inport  Port=2
  Constant4 : Constant  Value=0
  Switch1 : Switch  Criteria=u2 > Threshold
  Out1 : Outport
  wires:
  Constant4/1 -> Switch1/3
  switch/1 -> Switch1/2
  Switch1/1 -> Out1/1
  zt3/1 -> Switch1/1

== system chap05/Subsystem16/Subsystem1/Subsystem3/Subsystem2/Subsystem ==
  In1 : Inport
  switch : Inport  Port=2
  Constant1 : Constant  Value=0
  Constant2 : Constant  Value=0
  Discrete-Time Integrator2 : DiscreteIntegrator  gainval=1  InitialCondition=0.1  SampleTime=-1  ICPrevOutput=DiscIntNeverNeededParam  ICPrevScaledInput=DiscIntNeverNeededParam
  Switch : Switch  Criteria=u2 > Threshold
  Switch1 : Switch  Criteria=u2 > Threshold
  Out1 : Outport
  wires:
  switch/1 -> Switch/2, Switch1/2
  Switch1/1 -> Out1/1
  Constant2/1 -> Switch1/3
  Constant1/1 -> Switch/3
  Discrete-Time Integrator2/1 -> Switch1/1
  In1/1 -> Switch/1
  Switch/1 -> Discrete-Time Integrator2/1

== system chap05/Subsystem16/Subsystem1/Subsystem5/Subsystem/Subsystem ==
  zt3 : Inport
  switch : Inport  Port=2
  Constant4 : Constant  Value=0
  Switch1 : Switch  Criteria=u2 > Threshold
  Out1 : Outport
  wires:
  Constant4/1 -> Switch1/3
  switch/1 -> Switch1/2
  Switch1/1 -> Out1/1
  zt3/1 -> Switch1/1

== system chap05/Subsystem16/Subsystem1/Subsystem9/Subsystem/Subsystem ==
  zt3 : Inport
  switch : Inport  Port=2
  Constant4 : Constant  Value=0
  Switch1 : Switch  Criteria=u2 > Threshold
  Out1 : Outport
  wires:
  Constant4/1 -> Switch1/3
  switch/1 -> Switch1/2
  Switch1/1 -> Out1/1
  zt3/1 -> Switch1/1

== system chap05/Subsystem16/Subsystem2/Subsystem11/Subsystem/Subsystem ==
  zt3 : Inport
  switch : Inport  Port=2
  Constant4 : Constant  Value=0
  Switch1 : Switch  Criteria=u2 > Threshold
  Out1 : Outport
  wires:
  Constant4/1 -> Switch1/3
  switch/1 -> Switch1/2
  Switch1/1 -> Out1/1
  zt3/1 -> Switch1/1

== system chap05/Subsystem16/Subsystem2/Subsystem3/Subsystem2/Subsystem ==
  In1 : Inport
  switch : Inport  Port=2
  Constant1 : Constant  Value=0
  Constant2 : Constant  Value=0
  Discrete-Time Integrator2 : DiscreteIntegrator  gainval=1  InitialCondition=0.1  SampleTime=-1  ICPrevOutput=DiscIntNeverNeededParam  ICPrevScaledInput=DiscIntNeverNeededParam
  Switch : Switch  Criteria=u2 > Threshold
  Switch1 : Switch  Criteria=u2 > Threshold
  Out1 : Outport
  wires:
  switch/1 -> Switch/2, Switch1/2
  Switch1/1 -> Out1/1
  Constant2/1 -> Switch1/3
  Constant1/1 -> Switch/3
  Discrete-Time Integrator2/1 -> Switch1/1
  In1/1 -> Switch/1
  Switch/1 -> Discrete-Time Integrator2/1

== system chap05/Subsystem16/Subsystem2/Subsystem4/Subsystem/Subsystem ==
  zt3 : Inport
  switch : Inport  Port=2
  Constant4 : Constant  Value=0
  Switch1 : Switch  Criteria=u2 > Threshold
  Out1 : Outport
  wires:
  Constant4/1 -> Switch1/3
  switch/1 -> Switch1/2
  Switch1/1 -> Out1/1
  zt3/1 -> Switch1/1

== system chap05/Subsystem16/Subsystem2/Subsystem9/Subsystem/Subsystem ==
  zt3 : Inport
  switch : Inport  Port=2
  Constant4 : Constant  Value=0
  Switch1 : Switch  Criteria=u2 > Threshold
  Out1 : Outport
  wires:
  Constant4/1 -> Switch1/3
  switch/1 -> Switch1/2
  Switch1/1 -> Out1/1
  zt3/1 -> Switch1/1

== system chap05/Subsystem16/Subsystem3/Subsystem11/Subsystem/Subsystem ==
  zt3 : Inport
  switch : Inport  Port=2
  Constant4 : Constant  Value=0
  Switch1 : Switch  Criteria=u2 > Threshold
  Out1 : Outport
  wires:
  Constant4/1 -> Switch1/3
  switch/1 -> Switch1/2
  Switch1/1 -> Out1/1
  zt3/1 -> Switch1/1

== system chap05/Subsystem16/Subsystem3/Subsystem3/Subsystem2/Subsystem ==
  In1 : Inport
  switch : Inport  Port=2
  Constant1 : Constant  Value=0
  Constant2 : Constant  Value=0
  Discrete-Time Integrator2 : DiscreteIntegrator  gainval=1  InitialCondition=0.1  SampleTime=-1  ICPrevOutput=DiscIntNeverNeededParam  ICPrevScaledInput=DiscIntNeverNeededParam
  Switch : Switch  Criteria=u2 > Threshold
  Switch1 : Switch  Criteria=u2 > Threshold
  Out1 : Outport
  wires:
  switch/1 -> Switch/2, Switch1/2
  Switch1/1 -> Out1/1
  Constant2/1 -> Switch1/3
  Constant1/1 -> Switch/3
  Discrete-Time Integrator2/1 -> Switch1/1
  In1/1 -> Switch/1
  Switch/1 -> Discrete-Time Integrator2/1

== system chap05/Subsystem16/Subsystem3/Subsystem4/Subsystem/Subsystem ==
  zt3 : Inport
  switch : Inport  Port=2
  Constant4 : Constant  Value=0
  Switch1 : Switch  Criteria=u2 > Threshold
  Out1 : Outport
  wires:
  Constant4/1 -> Switch1/3
  switch/1 -> Switch1/2
  Switch1/1 -> Out1/1
  zt3/1 -> Switch1/1

== system chap05/Subsystem16/Subsystem3/Subsystem9/Subsystem/Subsystem ==
  zt3 : Inport
  switch : Inport  Port=2
  Constant4 : Constant  Value=0
  Switch1 : Switch  Criteria=u2 > Threshold
  Out1 : Outport
  wires:
  Constant4/1 -> Switch1/3
  switch/1 -> Switch1/2
  Switch1/1 -> Out1/1
  zt3/1 -> Switch1/1

== system chap05/Subsystem16/Subsystem5/Subsystem11/Subsystem/Subsystem ==
  zt3 : Inport
  switch : Inport  Port=2
  Constant4 : Constant  Value=0
  Switch1 : Switch  Criteria=u2 > Threshold
  Out1 : Outport
  wires:
  Constant4/1 -> Switch1/3
  switch/1 -> Switch1/2
  Switch1/1 -> Out1/1
  zt3/1 -> Switch1/1

== system chap05/Subsystem16/Subsystem5/Subsystem3/Subsystem2/Subsystem ==
  In1 : Inport
  switch : Inport  Port=2
  Constant1 : Constant  Value=0
  Constant2 : Constant  Value=0
  Discrete-Time Integrator2 : DiscreteIntegrator  gainval=1  InitialCondition=0.1  SampleTime=-1  ICPrevOutput=DiscIntNeverNeededParam  ICPrevScaledInput=DiscIntNeverNeededParam
  Switch : Switch  Criteria=u2 > Threshold
  Switch1 : Switch  Criteria=u2 > Threshold
  Out1 : Outport
  wires:
  switch/1 -> Switch/2, Switch1/2
  Switch1/1 -> Out1/1
  Constant2/1 -> Switch1/3
  Constant1/1 -> Switch/3
  Discrete-Time Integrator2/1 -> Switch1/1
  In1/1 -> Switch/1
  Switch/1 -> Discrete-Time Integrator2/1

== system chap05/Subsystem16/Subsystem5/Subsystem4/Subsystem/Subsystem ==
  zt3 : Inport
  switch : Inport  Port=2
  Constant4 : Constant  Value=0
  Switch1 : Switch  Criteria=u2 > Threshold
  Out1 : Outport
  wires:
  Constant4/1 -> Switch1/3
  switch/1 -> Switch1/2
  Switch1/1 -> Out1/1
  zt3/1 -> Switch1/1

== system chap05/Subsystem16/Subsystem5/Subsystem9/Subsystem/Subsystem ==
  zt3 : Inport
  switch : Inport  Port=2
  Constant4 : Constant  Value=0
  Switch1 : Switch  Criteria=u2 > Threshold
  Out1 : Outport
  wires:
  Constant4/1 -> Switch1/3
  switch/1 -> Switch1/2
  Switch1/1 -> Out1/1
  zt3/1 -> Switch1/1

== system chap05/Subsystem16/Subsystem6/Subsystem3/Subsystem2/Subsystem ==
  In1 : Inport
  switch : Inport  Port=2
  Constant1 : Constant  Value=0
  Constant2 : Constant  Value=0
  Discrete-Time Integrator2 : DiscreteIntegrator  gainval=1  InitialCondition=0.1  SampleTime=-1  ICPrevOutput=DiscIntNeverNeededParam  ICPrevScaledInput=DiscIntNeverNeededParam
  Switch : Switch  Criteria=u2 > Threshold
  Switch1 : Switch  Criteria=u2 > Threshold
  Out1 : Outport
  wires:
  switch/1 -> Switch/2, Switch1/2
  Switch1/1 -> Out1/1
  Constant2/1 -> Switch1/3
  Constant1/1 -> Switch/3
  Discrete-Time Integrator2/1 -> Switch1/1
  In1/1 -> Switch/1
  Switch/1 -> Discrete-Time Integrator2/1

== system chap05/Subsystem16/Subsystem6/Subsystem4/Subsystem/Subsystem ==
  zt3 : Inport
  switch : Inport  Port=2
  Constant4 : Constant  Value=0
  Switch1 : Switch  Criteria=u2 > Threshold
  Out1 : Outport
  wires:
  Constant4/1 -> Switch1/3
  switch/1 -> Switch1/2
  Switch1/1 -> Out1/1
  zt3/1 -> Switch1/1

== system chap05/Subsystem16/Subsystem6/Subsystem5/Subsystem/Subsystem ==
  zt3 : Inport
  switch : Inport  Port=2
  Constant4 : Constant  Value=0
  Switch1 : Switch  Criteria=u2 > Threshold
  Out1 : Outport
  wires:
  Constant4/1 -> Switch1/3
  switch/1 -> Switch1/2
  Switch1/1 -> Out1/1
  zt3/1 -> Switch1/1

== system chap05/Subsystem16/Subsystem6/Subsystem7/Subsystem/Subsystem ==
  zt3 : Inport
  switch : Inport  Port=2
  Constant4 : Constant  Value=0
  Switch1 : Switch  Criteria=u2 > Threshold
  Out1 : Outport
  wires:
  Constant4/1 -> Switch1/3
  switch/1 -> Switch1/2
  Switch1/1 -> Out1/1
  zt3/1 -> Switch1/1

== matlab function chap05/Subsystem16/Subsystem5/Subsystem3/Subsystem2/MATLAB Function ==
  data: u input; y output
function y = fcn(u)

y = norm(u);

== matlab function chap05/Subsystem16/Subsystem3/Subsystem3/Subsystem2/MATLAB Function ==
  data: u input; y output
function y = fcn(u)

y = norm(u);

== matlab function chap05/Subsystem16/Subsystem1/Subsystem3/Subsystem2/MATLAB Function ==
  data: u input; y output
function y = fcn(u)

y = norm(u);

== matlab function chap05/Subsystem16/Subsystem6/Subsystem3/Subsystem2/MATLAB Function ==
  data: u input; y output
function y = fcn(u)

y = norm(u);

== matlab function chap05/Subsystem16/Subsystem/Subsystem10/MATLAB Function ==
  data: u input; utk input; nrom output
function nrom = fcn(u,utk)

e = utk-u;
nrom = norm(e);

== matlab function chap05/Subsystem16/Subsystem1/Subsystem8/MATLAB Function ==
  data: u input; y output
function y = fcn(u)

y = norm(u);

== matlab function chap05/Subsystem16/Subsystem/Subsystem11/Subsystem/MATLAB Function ==
  data: u1 input; y output; u2 input
function y = fcn(u1,u2)


if (u1==u2)
    y = 0;
else
    y = 1;
end

== matlab function chap05/Subsystem16/Subsystem/Subsystem3/MATLAB Function ==
  data: u input; y output
function y = fcn(u)

y = u;

if y==0
    y=10e-15;
end

== matlab function chap05/Subsystem16/Subsystem/Subsystem3/MATLAB Function1 ==
  data: u input; y output
function y = fcn(u)

y = u;

if y==0
    y=10e-15;
end

== matlab function chap05/Subsystem16/Subsystem/Subsystem3/MATLAB Function2 ==
  data: u input; y output
function y = fcn(u)

y = u;

if y==0
    y=10e-15;
end

== matlab function chap05/Subsystem16/Subsystem/Subsystem3/Subsystem/MATLAB Function ==
  data: u input; y output
function y = fcn(u)

y = norm(u);

== matlab function chap05/Subsystem16/Subsystem/Subsystem3/Subsystem1/MATLAB Function ==
  data: u input; y output
function y = fcn(u)

y = norm(u)^(1/2);

== matlab function chap05/Subsystem16/Subsystem/Subsystem3/Subsystem2/MATLAB Function ==
  data: u input; y output
function y = fcn(u)

y = norm(u);

== matlab function chap05/Subsystem16/Subsystem/Subsystem4/Subsystem/MATLAB Function ==
  data: u1 input; y output; u2 input
function y = fcn(u1,u2)


if (u1==u2)
    y = 0;
else
    y = 1;
end

== matlab function chap05/Subsystem16/Subsystem/Subsystem9/Subsystem/MATLAB Function ==
  data: u1 input; y output; u2 input
function y = fcn(u1,u2)


if (u1==u2)
    y = 0;
else
    y = 1;
end

== matlab function chap05/Subsystem16/Subsystem1/Subsystem10/MATLAB Function ==
  data: u input; utk input; nrom output
function nrom = fcn(u,utk)

e = utk-u;
nrom = norm(e);

== matlab function chap05/Subsystem16/Subsystem6/Subsystem8/MATLAB Function ==
  data: u input; y output
function y = fcn(u)

y = norm(u);

== matlab function chap05/Subsystem16/Subsystem1/Subsystem3/MATLAB Function ==
  data: u input; y output
function y = fcn(u)

y = u;

if y==0
    y=10e-15;
end

== matlab function chap05/Subsystem16/Subsystem1/Subsystem3/MATLAB Function1 ==
  data: u input; y output
function y = fcn(u)

y = u;

if y==0
    y=10e-15;
end

== matlab function chap05/Subsystem16/Subsystem1/Subsystem3/MATLAB Function2 ==
  data: u input; y output
function y = fcn(u)

y = u;

if y==0
    y=10e-15;
end

== matlab function chap05/Subsystem16/Subsystem1/Subsystem3/Subsystem/MATLAB Function ==
  data: u input; y output
function y = fcn(u)

y = norm(u);

== matlab function chap05/Subsystem16/Subsystem1/Subsystem3/Subsystem1/MATLAB Function ==
  data: u input; y output
function y = fcn(u)

y = norm(u)^(1/2);

== matlab function chap05/Subsystem16/Subsystem3/Subsystem11/Subsystem/MATLAB Function ==
  data: u1 input; y output; u2 input
function y = fcn(u1,u2)


if (u1==u2)
    y = 0;
else
    y = 1;
end

== matlab function chap05/Subsystem16/Subsystem6/Subsystem10/MATLAB Function ==
  data: u input; utk input; nrom output
function nrom = fcn(u,utk)

e = utk-u;
nrom = norm(e);

== matlab function chap05/Subsystem16/Subsystem6/Subsystem3/MATLAB Function ==
  data: u input; y output
function y = fcn(u)

y = u;

if y==0
    y=10e-15;
end

== matlab function chap05/Subsystem16/Subsystem6/Subsystem3/MATLAB Function1 ==
  data: u input; y output
function y = fcn(u)

y = u;

if y==0
    y=10e-15;
end

== matlab function chap05/Subsystem16/Subsystem6/Subsystem8/MATLAB Function1 ==
  data: u input; y output
function y = fcn(u)

y = norm(u);

== matlab function chap05/Subsystem16/Subsystem6/Subsystem3/MATLAB Function2 ==
  data: u input; y output
function y = fcn(u)

y = u;

if y==0
    y=10e-15;
end

== matlab function chap05/Subsystem16/Subsystem6/Subsystem3/Subsystem/MATLAB Function ==
  data: u input; y output
function y = fcn(u)

y = norm(u);

== matlab function chap05/Subsystem16/Subsystem6/Subsystem3/Subsystem1/MATLAB Function ==
  data: u input; y output
function y = fcn(u)

y = norm(u)^(1/2);

== matlab function chap05/Subsystem16/Subsystem2/Subsystem10/MATLAB Function ==
  data: u input; utk input; nrom output
function nrom = fcn(u,utk)

e = utk-u;
nrom = norm(e);

== matlab function chap05/Subsystem16/Subsystem2/Subsystem11/Subsystem/MATLAB Function ==
  data: u1 input; y output; u2 input
function y = fcn(u1,u2)


if (u1==u2)
    y = 0;
else
    y = 1;
end

== matlab function chap05/Subsystem16/Subsystem2/Subsystem3/MATLAB Function ==
  data: u input; y output
function y = fcn(u)

y = u;

if y==0
    y=10e-15;
end

== matlab function chap05/Subsystem16/Subsystem2/Subsystem3/MATLAB Function1 ==
  data: u input; y output
function y = fcn(u)

y = u;

if y==0
    y=10e-15;
end

== matlab function chap05/Subsystem16/Subsystem2/Subsystem3/MATLAB Function2 ==
  data: u input; y output
function y = fcn(u)

y = u;

if y==0
    y=10e-15;
end

== matlab function chap05/Subsystem16/Subsystem2/Subsystem3/Subsystem/MATLAB Function ==
  data: u input; y output
function y = fcn(u)

y = norm(u);

== matlab function chap05/Subsystem16/Subsystem2/Subsystem3/Subsystem1/MATLAB Function ==
  data: u input; y output
function y = fcn(u)

y = norm(u)^(1/2);

== matlab function chap05/Subsystem16/Subsystem3/Subsystem8/MATLAB Function ==
  data: u input; y output
function y = fcn(u)

y = norm(u);

== matlab function chap05/Subsystem16/Subsystem2/Subsystem4/Subsystem/MATLAB Function ==
  data: u1 input; y output; u2 input
function y = fcn(u1,u2)


if (u1==u2)
    y = 0;
else
    y = 1;
end

== matlab function chap05/Subsystem16/Subsystem2/Subsystem9/Subsystem/MATLAB Function ==
  data: u1 input; y output; u2 input
function y = fcn(u1,u2)


if (u1==u2)
    y = 0;
else
    y = 1;
end

== matlab function chap05/Subsystem16/Subsystem3/Subsystem10/MATLAB Function ==
  data: u input; utk input; nrom output
function nrom = fcn(u,utk)

e = utk-u;
nrom = norm(e);

== matlab function chap05/Subsystem16/Subsystem3/Subsystem4/Subsystem/MATLAB Function ==
  data: u1 input; y output; u2 input
function y = fcn(u1,u2)


if (u1==u2)
    y = 0;
else
    y = 1;
end
